simulink model "inner_PD_thrust_d"  (R2018b)
settings: Solver=VariableStepAuto  StartTime=0.0  StopTime=10  RelTol=1e-3  EnableMultiTasking=on
settings Model: Creator=Daniel  LastModifiedBy=sstroobants
settings DataIOCC: LimitDataPoints=on
settings OptimizationCC: LifeSpan=inf
settings DebuggingCC: AllowSymbolicDim=off  SFUnexpectedBacktrackingDiag=warning  SFNoUnconditionalDefaultTransitionDiag=warning
settings ModelReferenceCC: PropagateSignalLabelsOutOfModel=off
settings SFSimCC: SimUseLocalCustomCode=off
settings RTWCC: RTWUseLocalCustomCode=off
settings CodeAppCC: StateflowObjectComments=on
settings GRTTargetCC: TargetLangStandard=C89/C90 (ANSI)
settings ConfigComp: CovMetricSettings=dw  CovHtmlReporting=on  CovSaveCumulativeToWorkspaceVar=on  CovSaveSingleToWorkspaceVar=on  CovExternalEMLEnable=off

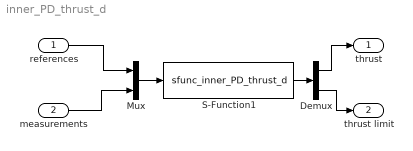
== system inner_PD_thrust_d ==
  references : Inport  PortDimensions=12
  measurements : Inport  Port=2  PortDimensions=12
  Demux : Demux  Outputs=2
  Mux : Mux  Inputs=2
  S-Function1 : S-Function  FunctionName=sfunc_inner_PD_thrust_d  Parameters=PD_thrust_param  SFunctionDeploymentMode=off  EnableBusSupport=off
  thrust : Outport
  thrust limit : Outport  Port=2
  wires:
  measurements/1 -> Mux/2
  references/1 -> Mux/1
  Mux/1 -> S-Function1/1
  S-Function1/1 -> Demux/1
  Demux/1 -> thrust/1
  Demux/2 -> thrust limit/1
